simulink model "sampleModel646original"  (R2021b)
settings: Solver=VariableStepAuto  StartTime=0.0  StopTime=10.0  RelTol=1e-3
undefined symbols (not defined in the file): DiscIntNeverNeededParam, Newton, Raphson, sigbuilder_block
libraries: simulink x194, slpidlib x27
(part 3 of 5)

== system sampleModel646original/emi_1578 ==
  In1 : Inport
  emi_1579 : Inport  Port=2
  emi_1581 : DeadZone  SaturateOnIntegerOverflow=on
  emi_1582 : DiscreteIntegrator  SampleTime=-1  ICPrevOutput=DiscIntNeverNeededParam  ICPrevScaledInput=DiscIntNeverNeededParam
  emi_{1583,1595,1598,1600} (4 alike) : simulink/Discontinuities/Saturation Dynamic  OutMin=[]  OutMax=[]  OutDataTypeStr=Inherit: Same as second input  OutDataType=fixdt(1, 16)  OutScaling=2^-10  DoSatur=off
  emi_1584 : Math  SaturateOnIntegerOverflow=on
  emi_1585 : Sqrt  Operator=rSqrt  SaturateOnIntegerOverflow=on
  emi_1586 : simulink/Discontinuities/Rate Limiter Dynamic
  emi_1587 : DiscreteFir
  emi_1588 : MinMax
  emi_1589 : simulink/Discrete/Discrete Derivative  gainval=1.0  ICPrevScaledInput=0.0  OutMin=[]  OutMax=[]  OutDataType=fixdt(1, 16)  OutScaling=2^-10  DoSatur=off
  emi_1590 : DiscreteFir
  emi_1591 : slpidlib/PID Controller  Controller=PID  Form=Parallel  TimeDomain=Discrete-time  UseExternalTs=off  SampleTime=-1  IntegratorMethod=Forward Euler  FilterMethod=Forward Euler  ControllerParametersSource=internal  P=1  I=1  D=0  UseFilter=on  N=100  TunerSelectOption=Transfer Function Based (PID Tuner App)  InitialConditionSource=internal  InitialConditionForIntegrator=0  InitialConditionForFilter=0  DifferentiatorICPrevScaledInput=0  ExternalReset=none  TrackingMode=off  Kt=1  LimitOutput=off  SatLimitsSource=internal  UpperSaturationLimit=inf  LowerSaturationLimit=-inf  LinearizeAsGain=off  AntiWindupMode=none  Kb=1  POutMin=[]  POutMax=[]  IOutMin=[]  IOutMax=[]  DOutMin=[]  DOutMax=[]  NOutMin=[]  NOutMax=[]  SumOutMin=[]  SumOutMax=[]  SaturationOutMin=[]  SaturationOutMax=[]  PParamMin=[]  PParamMax=[]  IParamMin=[]  IParamMax=[]  DParamMin=[]  DParamMax=[]  NParamMin=[]  NParamMax=[]  KbParamMin=[]  KbParamMax=[]  KtParamMin=[]  KtParamMax=[]  KbOutMin=[]  KbOutMax=[]  KtOutMin=[]  KtOutMax=[]  IntegratorOutMin=[]  IntegratorOutMax=[]  FilterOutMin=[]  FilterOutMax=[]  SumI1OutMin=[]  SumI1OutMax=[]  SumI2OutMin=[]  SumI2OutMax=[]  SumI3OutMin=[]  SumI3OutMax=[]  SumI4OutMin=[]  SumI4OutMax=[]  SumDOutMin=[]  SumDOutMax=[]  DifferentiatorOutMin=[]  DifferentiatorOutMax=[]  FilterDiffOutCoefMin=[]  FilterDiffOutCoefMax=[]  ReciprocalOutMin=[]  ReciprocalOutMax=[]  SumDenOutMin=[]  SumDenOutMax=[]  SumNumOutMin=[]  SumNumOutMax=[]  DivideOutMin=[]  DivideOutMax=[]  UdiffTsProdOutMin=[]  UdiffTsProdOutMax=[]  NTsProdOutMin=[]  NTsProdOutMax=[]  UintegralTsProdOutMin=[]  UintegralTsProdOutMax=[]  UngainTsProdOutMin=[]  UngainTsProdOutMax=[]  IntegratorContinuousStateAttributes=''  IntegratorStateMustResolveToSignalObject=off  IntegratorRTWStateStorageClass=Auto  FilterContinuousStateAttributes=''  FilterStateMustResolveToSignalObject=off  FilterRTWStateStorageClass=Auto  ParallelPVariant=InternalParameters  IdealPVariant=Disabled  IVariant=InternalParameters  DVariant=InternalParameters  IntegratorVariant=Discrete  SatVariant=Disabled  AWVariant=Passthrough  PCopyVariant=Disabled  TRVariant=Disabled  FdbkBlocksVariant=Forward  IdealPFdbkVariant=Disabled  SatFdbkVariant=Disabled  DerivativeFilterVariant=ForwardEulerFilter  NVariant=InternalParameters  NCopyVariant=Disabled  FilterICVariant=InternalICsFilter  IntegratorICVariant=InternalICs  ExternalResetVariant=Disabled  TRSumVariant=Passthrough  SumFdbkVariant=Disabled  SumVariant=Sum_PID  TsampFilterVariant=InternalTs  TsampNgainVariant=Passthrough  TsampIntegralVariant=Passthrough  ExternalSaturationOutDataTypeStr=Inherit: Same as second input
  emi_1592 : simulink/Discrete/Difference  ICPrevInput=0.0  OutMin=[]  OutMax=[]  OutDataType=fixdt(1, 16)  OutScaling=2^-10  DoSatur=off
  emi_1593 : Trigonometry
  emi_1594 : Sum  Inputs=+
  emi_1596 : Product  Inputs=*
  emi_1597 : Sum  Inputs=+
  emi_1599 : RateLimiter  SampleTimeMode=inherited
  emi_1601 : DiscreteIntegrator  SampleTime=-1  ICPrevOutput=DiscIntNeverNeededParam  ICPrevScaledInput=DiscIntNeverNeededParam
  emi_1602 : simulink/Discrete/Transfer Fcn First Order  PoleZ=0.95  ICPrevOutput=0.0  DoSatur=off
  emi_1603 : Gain
  emi_1604 : simulink/Discontinuities/Rate Limiter Dynamic
  emi_1605 : DiscreteTransferFcn
  emi_1606 : simulink/Discrete/Discrete Derivative  gainval=1.0  ICPrevScaledInput=0.0  OutMin=[]  OutMax=[]  OutDataType=fixdt(1, 16)  OutScaling=2^-10  DoSatur=off
  emi_1607 : Clock
  Out1 : Outport
  emi_1580 : Outport  Port=2
  wires:
  In1/1 -> Out1/1
  emi_1581/1 -> emi_1582/1
  emi_1582/1 -> emi_1583/1
  emi_1583/1 -> emi_1584/1
  emi_1584/1 -> emi_1585/1
  emi_1585/1 -> emi_1586/1
  emi_1586/1 -> emi_1587/1
  emi_1587/1 -> emi_1588/1
  emi_1588/1 -> emi_1589/1
  emi_1589/1 -> emi_1590/1
  emi_1590/1 -> emi_1591/1
  emi_1591/1 -> emi_1592/1
  emi_1592/1 -> emi_1593/1
  emi_1593/1 -> emi_1594/1
  emi_1594/1 -> emi_1595/1
  emi_1595/1 -> emi_1596/1
  emi_1596/1 -> emi_1597/1
  emi_1597/1 -> emi_1598/1
  emi_1598/1 -> emi_1599/1
  emi_1599/1 -> emi_1600/1
  emi_1600/1 -> emi_1601/1
  emi_1601/1 -> emi_1602/1
  emi_1602/1 -> emi_1603/1
  emi_1603/1 -> emi_1604/1
  emi_1604/1 -> emi_1605/1
  emi_1605/1 -> emi_1606/1
  emi_1607/1 -> emi_1581/1
  emi_1606/1 -> emi_1580/1

== system sampleModel646original/emi_1614 ==
  emi_1621 : Inport
  Action Port : ActionPort  ActionPortLabel=if(0 > u1)
  emi_1618 : Trigonometry  SampleTime=1
  emi_1619 : Gain  SampleTime=1
  emi_1620 : Gain  SampleTime=1
  emi_{1623,1627,1638,1644,1646} (5 alike) : Sin  TimeSource=Use external signal  SampleTime=0
  emi_1624 : Math  SaturateOnIntegerOverflow=on
  emi_1625 : Rounding
  emi_{1626,1632,1640,1642,1650..1651,1653} (7 alike) : Sum  Inputs=+
  emi_1628 : MinMax
  emi_1629 : Sqrt  Operator=rSqrt  SaturateOnIntegerOverflow=on
  emi_1630 : UnaryMinus
  emi_1631 : Product  Inputs=*
  emi_1633 : MinMax
  emi_1634 : Product  Inputs=*
  emi_1635 : Gain
  emi_1636 : Trigonometry
  emi_1637 : Abs
  emi_1639 : Product  Inputs=*
  emi_1641 : Math  SaturateOnIntegerOverflow=on
  emi_1643 : UnaryMinus
  emi_1645 : Trigonometry
  emi_1647 : Rounding
  emi_1648 : Trigonometry
  emi_1649 : MinMax
  emi_1652 : Math  SaturateOnIntegerOverflow=on
  emi_1654 : Sqrt  Operator=rSqrt  SaturateOnIntegerOverflow=on
  emi_1655 : Ground
  emi_1622 : Outport
  wires:
  emi_1621/1 -> emi_1618/1
  emi_1618/1 -> emi_1619/1
  emi_1619/1 -> emi_1620/1
  emi_1623/1 -> emi_1624/1
  emi_1624/1 -> emi_1625/1
  emi_1625/1 -> emi_1626/1
  emi_1626/1 -> emi_1627/1
  emi_1627/1 -> emi_1628/1
  emi_1628/1 -> emi_1629/1
  emi_1629/1 -> emi_1630/1
  emi_1630/1 -> emi_1631/1
  emi_1631/1 -> emi_1632/1
  emi_1632/1 -> emi_1633/1
  emi_1633/1 -> emi_1634/1
  emi_1634/1 -> emi_1635/1
  emi_1635/1 -> emi_1636/1
  emi_1636/1 -> emi_1637/1
  emi_1637/1 -> emi_1638/1
  emi_1638/1 -> emi_1639/1
  emi_1639/1 -> emi_1640/1
  emi_1640/1 -> emi_1641/1
  emi_1641/1 -> emi_1642/1
  emi_1642/1 -> emi_1643/1
  emi_1643/1 -> emi_1644/1
  emi_1644/1 -> emi_1645/1
  emi_1645/1 -> emi_1646/1
  emi_1646/1 -> emi_1647/1
  emi_1647/1 -> emi_1648/1
  emi_1648/1 -> emi_1649/1
  emi_1649/1 -> emi_1650/1
  emi_1650/1 -> emi_1651/1
  emi_1651/1 -> emi_1652/1
  emi_1652/1 -> emi_1653/1
  emi_1653/1 -> emi_1654/1
  emi_1655/1 -> emi_1623/1
  emi_1654/1 -> emi_1622/1

== system sampleModel646original/emi_1658 ==
  In1 : Inport
  emi_1659 : Inport  Port=2
  emi_1661 : Trigonometry
  emi_1662 : Math  SaturateOnIntegerOverflow=on
  emi_1663 : simulink/Discrete/Difference  ICPrevInput=0.0  OutMin=[]  OutMax=[]  OutDataType=fixdt(1, 16)  OutScaling=2^-10  DoSatur=off
  emi_{1664,1679,1682,1691} (4 alike) : simulink/Discrete/Discrete Derivative  gainval=1.0  ICPrevScaledInput=0.0  OutMin=[]  OutMax=[]  OutDataType=fixdt(1, 16)  OutScaling=2^-10  DoSatur=off
  emi_1665 : DiscreteIntegrator  SampleTime=-1  ICPrevOutput=DiscIntNeverNeededParam  ICPrevScaledInput=DiscIntNeverNeededParam
  emi_1666 : RateLimiter  SampleTimeMode=inherited
  emi_1667 : slpidlib/PID Controller  Controller=PID  Form=Parallel  TimeDomain=Discrete-time  UseExternalTs=off  SampleTime=-1  IntegratorMethod=Forward Euler  FilterMethod=Forward Euler  ControllerParametersSource=internal  P=1  I=1  D=0  UseFilter=on  N=100  TunerSelectOption=Transfer Function Based (PID Tuner App)  InitialConditionSource=internal  InitialConditionForIntegrator=0  InitialConditionForFilter=0  DifferentiatorICPrevScaledInput=0  ExternalReset=none  TrackingMode=off  Kt=1  LimitOutput=off  SatLimitsSource=internal  UpperSaturationLimit=inf  LowerSaturationLimit=-inf  LinearizeAsGain=off  AntiWindupMode=none  Kb=1  POutMin=[]  POutMax=[]  IOutMin=[]  IOutMax=[]  DOutMin=[]  DOutMax=[]  NOutMin=[]  NOutMax=[]  SumOutMin=[]  SumOutMax=[]  SaturationOutMin=[]  SaturationOutMax=[]  PParamMin=[]  PParamMax=[]  IParamMin=[]  IParamMax=[]  DParamMin=[]  DParamMax=[]  NParamMin=[]  NParamMax=[]  KbParamMin=[]  KbParamMax=[]  KtParamMin=[]  KtParamMax=[]  KbOutMin=[]  KbOutMax=[]  KtOutMin=[]  KtOutMax=[]  IntegratorOutMin=[]  IntegratorOutMax=[]  FilterOutMin=[]  FilterOutMax=[]  SumI1OutMin=[]  SumI1OutMax=[]  SumI2OutMin=[]  SumI2OutMax=[]  SumI3OutMin=[]  SumI3OutMax=[]  SumI4OutMin=[]  SumI4OutMax=[]  SumDOutMin=[]  SumDOutMax=[]  DifferentiatorOutMin=[]  DifferentiatorOutMax=[]  FilterDiffOutCoefMin=[]  FilterDiffOutCoefMax=[]  ReciprocalOutMin=[]  ReciprocalOutMax=[]  SumDenOutMin=[]  SumDenOutMax=[]  SumNumOutMin=[]  SumNumOutMax=[]  DivideOutMin=[]  DivideOutMax=[]  UdiffTsProdOutMin=[]  UdiffTsProdOutMax=[]  NTsProdOutMin=[]  NTsProdOutMax=[]  UintegralTsProdOutMin=[]  UintegralTsProdOutMax=[]  UngainTsProdOutMin=[]  UngainTsProdOutMax=[]  IntegratorContinuousStateAttributes=''  IntegratorStateMustResolveToSignalObject=off  IntegratorRTWStateStorageClass=Auto  FilterContinuousStateAttributes=''  FilterStateMustResolveToSignalObject=off  FilterRTWStateStorageClass=Auto  ParallelPVariant=InternalParameters  IdealPVariant=Disabled  IVariant=InternalParameters  DVariant=InternalParameters  IntegratorVariant=Discrete  SatVariant=Disabled  AWVariant=Passthrough  PCopyVariant=Disabled  TRVariant=Disabled  FdbkBlocksVariant=Forward  IdealPFdbkVariant=Disabled  SatFdbkVariant=Disabled  DerivativeFilterVariant=ForwardEulerFilter  NVariant=InternalParameters  NCopyVariant=Disabled  FilterICVariant=InternalICsFilter  IntegratorICVariant=InternalICs  ExternalResetVariant=Disabled  TRSumVariant=Passthrough  SumFdbkVariant=Disabled  SumVariant=Sum_PID  TsampFilterVariant=InternalTs  TsampNgainVariant=Passthrough  TsampIntegralVariant=Passthrough  ExternalSaturationOutDataTypeStr=Inherit: Same as second input
  emi_1668 : Sqrt  Operator=rSqrt  SaturateOnIntegerOverflow=on
  emi_1669 : simulink/Discontinuities/Rate Limiter Dynamic
  emi_1670 : slpidlib/PID Controller  Controller=PID  Form=Parallel  TimeDomain=Discrete-time  UseExternalTs=off  SampleTime=-1  IntegratorMethod=Forward Euler  FilterMethod=Forward Euler  ControllerParametersSource=internal  P=1  I=1  D=0  UseFilter=on  N=100  TunerSelectOption=Transfer Function Based (PID Tuner App)  InitialConditionSource=internal  InitialConditionForIntegrator=0  InitialConditionForFilter=0  DifferentiatorICPrevScaledInput=0  ExternalReset=none  TrackingMode=off  Kt=1  LimitOutput=off  SatLimitsSource=internal  UpperSaturationLimit=inf  LowerSaturationLimit=-inf  LinearizeAsGain=off  AntiWindupMode=none  Kb=1  POutMin=[]  POutMax=[]  IOutMin=[]  IOutMax=[]  DOutMin=[]  DOutMax=[]  NOutMin=[]  NOutMax=[]  SumOutMin=[]  SumOutMax=[]  SaturationOutMin=[]  SaturationOutMax=[]  PParamMin=[]  PParamMax=[]  IParamMin=[]  IParamMax=[]  DParamMin=[]  DParamMax=[]  NParamMin=[]  NParamMax=[]  KbParamMin=[]  KbParamMax=[]  KtParamMin=[]  KtParamMax=[]  KbOutMin=[]  KbOutMax=[]  KtOutMin=[]  KtOutMax=[]  IntegratorOutMin=[]  IntegratorOutMax=[]  FilterOutMin=[]  FilterOutMax=[]  SumI1OutMin=[]  SumI1OutMax=[]  SumI2OutMin=[]  SumI2OutMax=[]  SumI3OutMin=[]  SumI3OutMax=[]  SumI4OutMin=[]  SumI4OutMax=[]  SumDOutMin=[]  SumDOutMax=[]  DifferentiatorOutMin=[]  DifferentiatorOutMax=[]  FilterDiffOutCoefMin=[]  FilterDiffOutCoefMax=[]  ReciprocalOutMin=[]  ReciprocalOutMax=[]  SumDenOutMin=[]  SumDenOutMax=[]  SumNumOutMin=[]  SumNumOutMax=[]  DivideOutMin=[]  DivideOutMax=[]  UdiffTsProdOutMin=[]  UdiffTsProdOutMax=[]  NTsProdOutMin=[]  NTsProdOutMax=[]  UintegralTsProdOutMin=[]  UintegralTsProdOutMax=[]  UngainTsProdOutMin=[]  UngainTsProdOutMax=[]  IntegratorContinuousStateAttributes=''  IntegratorStateMustResolveToSignalObject=off  IntegratorRTWStateStorageClass=Auto  FilterContinuousStateAttributes=''  FilterStateMustResolveToSignalObject=off  FilterRTWStateStorageClass=Auto  ParallelPVariant=InternalParameters  IdealPVariant=Disabled  IVariant=InternalParameters  DVariant=InternalParameters  IntegratorVariant=Discrete  SatVariant=Disabled  AWVariant=Passthrough  PCopyVariant=Disabled  TRVariant=Disabled  FdbkBlocksVariant=Forward  IdealPFdbkVariant=Disabled  SatFdbkVariant=Disabled  DerivativeFilterVariant=ForwardEulerFilter  NVariant=InternalParameters  NCopyVariant=Disabled  FilterICVariant=InternalICsFilter  IntegratorICVariant=InternalICs  ExternalResetVariant=Disabled  TRSumVariant=Passthrough  SumFdbkVariant=Disabled  SumVariant=Sum_PID  TsampFilterVariant=InternalTs  TsampNgainVariant=Passthrough  TsampIntegralVariant=Passthrough  ExternalSaturationOutDataTypeStr=Inherit: Same as second input
  emi_1671 : simulink/Discrete/Difference  ICPrevInput=0.0  OutMin=[]  OutMax=[]  OutDataType=fixdt(1, 16)  OutScaling=2^-10  DoSatur=off
  emi_1672 : Math  SaturateOnIntegerOverflow=on
  emi_1673 : Rounding
  emi_1674 : simulink/Discrete/Transfer Fcn First Order  PoleZ=0.95  ICPrevOutput=0.0  DoSatur=off
  emi_1675 : Relay
  emi_1676 : Rounding
  emi_1677 : simulink/Discontinuities/PWM  DisableCoverage=on  Period=1  DisallowZeroDutyCycle=off  RunAtFixedTimeIntervals=off  SampleTime=0.1
  emi_1678 : Sum  Inputs=+
  emi_1680 : simulink/Discontinuities/Saturation Dynamic  OutMin=[]  OutMax=[]  OutDataTypeStr=Inherit: Same as second input  OutDataType=fixdt(1, 16)  OutScaling=2^-10  DoSatur=off
  emi_1681 : Gain
  emi_1683 : RateLimiter  SampleTimeMode=inherited
  emi_1684 : DiscreteFir
  emi_1685 : DeadZone  SaturateOnIntegerOverflow=on
  emi_1686 : simulink/Discontinuities/PWM  DisableCoverage=on  Period=1  DisallowZeroDutyCycle=off  RunAtFixedTimeIntervals=off  SampleTime=0.1
  emi_1687 : Sin  TimeSource=Use external signal  SampleTime=0
  emi_1688 : Quantizer
  emi_1689 : RateLimiter  SampleTimeMode=inherited
  emi_1690 : DiscreteZeroPole  Poles=[0 0.5]  Gain=1  SampleTime=-1
  emi_1692 : simulink/Discontinuities/Wrap To Zero  Threshold=255
      settings: SourceProductBaseCode=SL
  emi_1693 : simulink/Sources/Repeating Sequence  rep_seq_t=[0 2]  rep_seq_y=[0 2]
  Out1 : Outport
  emi_1660 : Outport  Port=2
  wires:
  In1/1 -> Out1/1
  emi_1661/1 -> emi_1662/1
  emi_1662/1 -> emi_1663/1
  emi_1663/1 -> emi_1664/1
  emi_1664/1 -> emi_1665/1
  emi_1665/1 -> emi_1666/1
  emi_1666/1 -> emi_1667/1
  emi_1667/1 -> emi_1668/1
  emi_1668/1 -> emi_1669/1
  emi_1669/1 -> emi_1670/1
  emi_1670/1 -> emi_1671/1
  emi_1671/1 -> emi_1672/1
  emi_1672/1 -> emi_1673/1
  emi_1673/1 -> emi_1674/1
  emi_1674/1 -> emi_1675/1
  emi_1675/1 -> emi_1676/1
  emi_1676/1 -> emi_1677/1
  emi_1677/1 -> emi_1678/1
  emi_1678/1 -> emi_1679/1
  emi_1679/1 -> emi_1680/1
  emi_1680/1 -> emi_1681/1
  emi_1681/1 -> emi_1682/1
  emi_1682/1 -> emi_1683/1
  emi_1683/1 -> emi_1684/1
  emi_1684/1 -> emi_1685/1
  emi_1685/1 -> emi_1686/1
  emi_1686/1 -> emi_1687/1
  emi_1687/1 -> emi_1688/1
  emi_1688/1 -> emi_1689/1
  emi_1689/1 -> emi_1690/1
  emi_1690/1 -> emi_1691/1
  emi_1691/1 -> emi_1692/1
  emi_1693/1 -> emi_1661/1
  emi_1692/1 -> emi_1660/1

== system sampleModel646original/emi_166 ==
  emi_173 : Inport
  Action Port : ActionPort  ActionPortLabel=if(0 > u1)
  emi_170 : MinMax  SampleTime=1
  emi_171 : Trigonometry  SampleTime=1
  emi_172 : Math  SampleTime=1  SaturateOnIntegerOverflow=on
  emi_175 : Trigonometry
  emi_176 : Gain
  emi_177 : Sin  TimeSource=Use external signal  SampleTime=0
  emi_178 : Sqrt  Operator=rSqrt  SaturateOnIntegerOverflow=on
  emi_179 : UnaryMinus
  emi_180 : Sqrt  Operator=rSqrt  SaturateOnIntegerOverflow=on
  emi_181 : Sum  Inputs=+
  emi_182 : MinMax
  emi_183 : Abs
  emi_184 : Sqrt  Operator=rSqrt  SaturateOnIntegerOverflow=on
  emi_185 : Math  SaturateOnIntegerOverflow=on
  emi_186 : UnaryMinus
  emi_187 : UnaryMinus
  emi_188 : Trigonometry
  emi_189 : Rounding
  emi_190 : Math  SaturateOnIntegerOverflow=on
  emi_191 : Gain
  emi_192 : Gain
  emi_193 : Abs
  emi_194 : Ground
  emi_174 : Outport
  wires:
  emi_173/1 -> emi_170/1
  emi_170/1 -> emi_171/1
  emi_171/1 -> emi_172/1
  emi_175/1 -> emi_176/1
  emi_176/1 -> emi_177/1
  emi_177/1 -> emi_178/1
  emi_178/1 -> emi_179/1
  emi_179/1 -> emi_180/1
  emi_180/1 -> emi_181/1
  emi_181/1 -> emi_182/1
  emi_182/1 -> emi_183/1
  emi_183/1 -> emi_184/1
  emi_184/1 -> emi_185/1
  emi_185/1 -> emi_186/1
  emi_186/1 -> emi_187/1
  emi_187/1 -> emi_188/1
  emi_188/1 -> emi_189/1
  emi_189/1 -> emi_190/1
  emi_190/1 -> emi_191/1
  emi_191/1 -> emi_192/1
  emi_192/1 -> emi_193/1
  emi_194/1 -> emi_175/1
  emi_193/1 -> emi_174/1

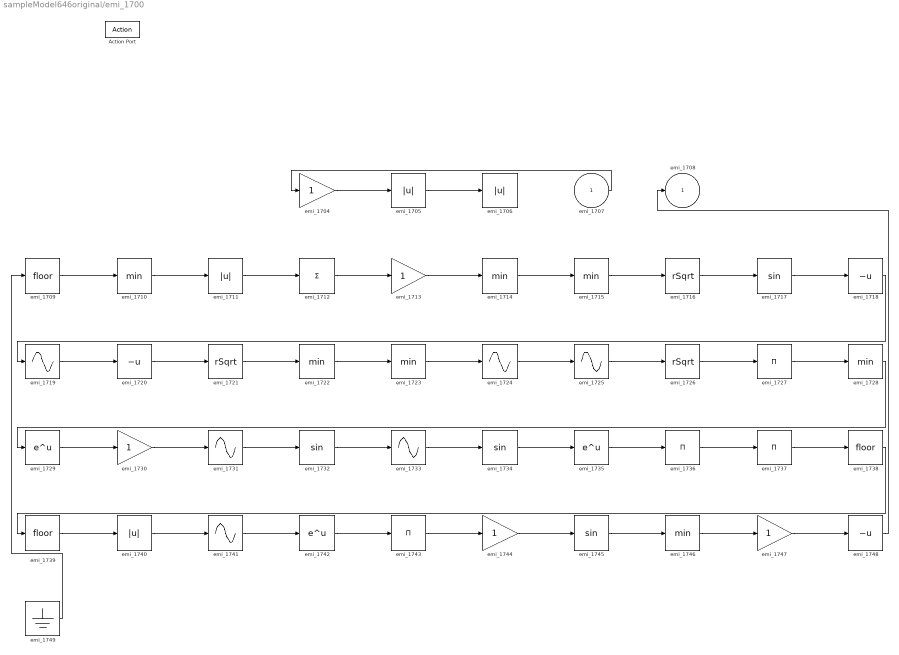
== system sampleModel646original/emi_1700 ==
  emi_1707 : Inport
  Action Port : ActionPort  ActionPortLabel=if(0 > u1)
  emi_{1704,1713,1730,1744,1747} (5 alike) : Gain
  emi_{1705..1706,1711,1740} (4 alike) : Abs
  emi_1709 : Rounding
  emi_{1710,1714..1715,1722..1723,1728,1746} (7 alike) : MinMax
  emi_1712 : Sum  Inputs=+
  emi_1716 : Sqrt  Operator=rSqrt  SaturateOnIntegerOverflow=on
  emi_{1717,1732,1734,1745} (4 alike) : Trigonometry
  emi_1718 : UnaryMinus
  emi_{1719,1724..1725,1731,1733,1741} (6 alike) : Sin  TimeSource=Use external signal  SampleTime=0
  emi_1720 : UnaryMinus
  emi_1721 : Sqrt  Operator=rSqrt  SaturateOnIntegerOverflow=on
  emi_1726 : Sqrt  Operator=rSqrt  SaturateOnIntegerOverflow=on
  emi_{1727,1736..1737,1743} (4 alike) : Product  Inputs=*
  emi_1729 : Math  SaturateOnIntegerOverflow=on
  emi_1735 : Math  SaturateOnIntegerOverflow=on
  emi_1738 : Rounding
  emi_1739 : Rounding
  emi_1742 : Math  SaturateOnIntegerOverflow=on
  emi_1748 : UnaryMinus
  emi_1749 : Ground
  emi_1708 : Outport
  wires:
  emi_1707/1 -> emi_1704/1
  emi_1704/1 -> emi_1705/1
  emi_1705/1 -> emi_1706/1
  emi_1709/1 -> emi_1710/1
  emi_1710/1 -> emi_1711/1
  emi_1711/1 -> emi_1712/1
  emi_1712/1 -> emi_1713/1
  emi_1713/1 -> emi_1714/1
  emi_1714/1 -> emi_1715/1
  emi_1715/1 -> emi_1716/1
  emi_1716/1 -> emi_1717/1
  emi_1717/1 -> emi_1718/1
  emi_1718/1 -> emi_1719/1
  emi_1719/1 -> emi_1720/1
  emi_1720/1 -> emi_1721/1
  emi_1721/1 -> emi_1722/1
  emi_1722/1 -> emi_1723/1
  emi_1723/1 -> emi_1724/1
  emi_1724/1 -> emi_1725/1
  emi_1725/1 -> emi_1726/1
  emi_1726/1 -> emi_1727/1
  emi_1727/1 -> emi_1728/1
  emi_1728/1 -> emi_1729/1
  emi_1729/1 -> emi_1730/1
  emi_1730/1 -> emi_1731/1
  emi_1731/1 -> emi_1732/1
  emi_1732/1 -> emi_1733/1
  emi_1733/1 -> emi_1734/1
  emi_1734/1 -> emi_1735/1
  emi_1735/1 -> emi_1736/1
  emi_1736/1 -> emi_1737/1
  emi_1737/1 -> emi_1738/1
  emi_1738/1 -> emi_1739/1
  emi_1739/1 -> emi_1740/1
  emi_1740/1 -> emi_1741/1
  emi_1741/1 -> emi_1742/1
  emi_1742/1 -> emi_1743/1
  emi_1743/1 -> emi_1744/1
  emi_1744/1 -> emi_1745/1
  emi_1745/1 -> emi_1746/1
  emi_1746/1 -> emi_1747/1
  emi_1747/1 -> emi_1748/1
  emi_1749/1 -> emi_1709/1
  emi_1748/1 -> emi_1708/1

== system sampleModel646original/emi_1752 ==
  In1 : Inport
  emi_1753 : Inport  Port=2
  emi_1755 : simulink/Discontinuities/Saturation Dynamic  OutMin=[]  OutMax=[]  OutDataTypeStr=Inherit: Same as second input  OutDataType=fixdt(1, 16)  OutScaling=2^-10  DoSatur=off
  emi_1756 : Trigonometry
  emi_1757 : simulink/Discontinuities/Rate Limiter Dynamic
  emi_1758 : Trigonometry
  emi_1759 : Sin  TimeSource=Use external signal  SampleTime=0
  emi_1760 : UnaryMinus
  emi_1761 : DiscreteFir
  emi_1762 : Relay
  emi_1763 : simulink/Discontinuities/PWM  DisableCoverage=on  Period=1  DisallowZeroDutyCycle=off  RunAtFixedTimeIntervals=off  SampleTime=0.1
  emi_1764 : simulink/Discontinuities/Wrap To Zero  Threshold=255
      settings: SourceProductBaseCode=SL
  emi_1765 : MinMax
  emi_1766 : Rounding
  emi_1767 : DiscreteStateSpace  SampleTime=-1
  emi_1768 : simulink/Discrete/Transfer Fcn First Order  PoleZ=0.95  ICPrevOutput=0.0  DoSatur=off
  emi_1769 : Quantizer
  emi_1770 : DiscreteTransferFcn
  emi_1771 : simulink/Discontinuities/PWM  DisableCoverage=on  Period=1  DisallowZeroDutyCycle=off  RunAtFixedTimeIntervals=off  SampleTime=0.1
  emi_1772 : simulink/Discontinuities/PWM  DisableCoverage=on  Period=1  DisallowZeroDutyCycle=off  RunAtFixedTimeIntervals=off  SampleTime=0.1
  emi_1773 : DiscretePulseGenerator  PulseType=Time based  Period=10  PulseWidth=5
  Out1 : Outport
  emi_1754 : Outport  Port=2
  wires:
  In1/1 -> Out1/1
  emi_1755/1 -> emi_1756/1
  emi_1756/1 -> emi_1757/1
  emi_1757/1 -> emi_1758/1
  emi_1758/1 -> emi_1759/1
  emi_1759/1 -> emi_1760/1
  emi_1760/1 -> emi_1761/1
  emi_1761/1 -> emi_1762/1
  emi_1762/1 -> emi_1763/1
  emi_1763/1 -> emi_1764/1
  emi_1764/1 -> emi_1765/1
  emi_1765/1 -> emi_1766/1
  emi_1766/1 -> emi_1767/1
  emi_1767/1 -> emi_1768/1
  emi_1768/1 -> emi_1769/1
  emi_1769/1 -> emi_1770/1
  emi_1770/1 -> emi_1771/1
  emi_1771/1 -> emi_1772/1
  emi_1773/1 -> emi_1755/1
  emi_1772/1 -> emi_1754/1

== system sampleModel646original/emi_1781 ==
  emi_1788 : Inport
  Action Port : ActionPort  ActionPortLabel=if(-2 > u1)
  emi_1785 : Gain
  emi_1786 : Gain
  emi_1787 : Math  SaturateOnIntegerOverflow=on
  emi_1790 : UnaryMinus
  emi_1791 : Rounding
  emi_{1792,1795,1798,1801} (4 alike) : Product  Inputs=*
  emi_1793 : Rounding
  emi_1794 : Gain
  emi_1796 : Sin  TimeSource=Use external signal  SampleTime=0
  emi_1797 : Trigonometry
  emi_1799 : Math  SaturateOnIntegerOverflow=on
  emi_1800 : Sqrt  Operator=rSqrt  SaturateOnIntegerOverflow=on
  emi_1802 : UnaryMinus
  emi_1803 : Trigonometry
  emi_1804 : Ground
  emi_1789 : Outport
  wires:
  emi_1788/1 -> emi_1785/1
  emi_1785/1 -> emi_1786/1
  emi_1786/1 -> emi_1787/1
  emi_1790/1 -> emi_1791/1
  emi_1791/1 -> emi_1792/1
  emi_1792/1 -> emi_1793/1
  emi_1793/1 -> emi_1794/1
  emi_1794/1 -> emi_1795/1
  emi_1795/1 -> emi_1796/1
  emi_1796/1 -> emi_1797/1
  emi_1797/1 -> emi_1798/1
  emi_1798/1 -> emi_1799/1
  emi_1799/1 -> emi_1800/1
  emi_1800/1 -> emi_1801/1
  emi_1801/1 -> emi_1802/1
  emi_1802/1 -> emi_1803/1
  emi_1804/1 -> emi_1790/1
  emi_1803/1 -> emi_1789/1

== system sampleModel646original/emi_1807 ==
  In1 : Inport
  emi_1808 : Inport  Port=2
  emi_{1810,1820,1827..1828} (4 alike) : Math  SaturateOnIntegerOverflow=on
  emi_1811 : DiscreteStateSpace  SampleTime=-1
  emi_1812 : DiscreteFir
  emi_1813 : simulink/Discrete/Difference  ICPrevInput=0.0  OutMin=[]  OutMax=[]  OutDataType=fixdt(1, 16)  OutScaling=2^-10  DoSatur=off
  emi_1814 : DeadZone  SaturateOnIntegerOverflow=on
  emi_1815 : VariablePulseGenerator  SampleTime=0.1
  emi_1816 : Sin  TimeSource=Use external signal  SampleTime=0
  emi_1817 : Sqrt  Operator=rSqrt  SaturateOnIntegerOverflow=on
  emi_1818 : Abs
  emi_1819 : DiscreteFir
  emi_1821 : simulink/Discontinuities/Wrap To Zero  Threshold=255
      settings: SourceProductBaseCode=SL
  emi_1822 : simulink/Discontinuities/PWM  DisableCoverage=on  Period=1  DisallowZeroDutyCycle=off  RunAtFixedTimeIntervals=off  SampleTime=0.1
  emi_1823 : DiscreteFir
  emi_1824 : Relay
  emi_1825 : Abs
  emi_1826 : Relay
  emi_1829 : slpidlib/PID Controller  Controller=PID  Form=Parallel  TimeDomain=Discrete-time  UseExternalTs=off  SampleTime=-1  IntegratorMethod=Forward Euler  FilterMethod=Forward Euler  ControllerParametersSource=internal  P=1  I=1  D=0  UseFilter=on  N=100  TunerSelectOption=Transfer Function Based (PID Tuner App)  InitialConditionSource=internal  InitialConditionForIntegrator=0  InitialConditionForFilter=0  DifferentiatorICPrevScaledInput=0  ExternalReset=none  TrackingMode=off  Kt=1  LimitOutput=off  SatLimitsSource=internal  UpperSaturationLimit=inf  LowerSaturationLimit=-inf  LinearizeAsGain=off  AntiWindupMode=none  Kb=1  POutMin=[]  POutMax=[]  IOutMin=[]  IOutMax=[]  DOutMin=[]  DOutMax=[]  NOutMin=[]  NOutMax=[]  SumOutMin=[]  SumOutMax=[]  SaturationOutMin=[]  SaturationOutMax=[]  PParamMin=[]  PParamMax=[]  IParamMin=[]  IParamMax=[]  DParamMin=[]  DParamMax=[]  NParamMin=[]  NParamMax=[]  KbParamMin=[]  KbParamMax=[]  KtParamMin=[]  KtParamMax=[]  KbOutMin=[]  KbOutMax=[]  KtOutMin=[]  KtOutMax=[]  IntegratorOutMin=[]  IntegratorOutMax=[]  FilterOutMin=[]  FilterOutMax=[]  SumI1OutMin=[]  SumI1OutMax=[]  SumI2OutMin=[]  SumI2OutMax=[]  SumI3OutMin=[]  SumI3OutMax=[]  SumI4OutMin=[]  SumI4OutMax=[]  SumDOutMin=[]  SumDOutMax=[]  DifferentiatorOutMin=[]  DifferentiatorOutMax=[]  FilterDiffOutCoefMin=[]  FilterDiffOutCoefMax=[]  ReciprocalOutMin=[]  ReciprocalOutMax=[]  SumDenOutMin=[]  SumDenOutMax=[]  SumNumOutMin=[]  SumNumOutMax=[]  DivideOutMin=[]  DivideOutMax=[]  UdiffTsProdOutMin=[]  UdiffTsProdOutMax=[]  NTsProdOutMin=[]  NTsProdOutMax=[]  UintegralTsProdOutMin=[]  UintegralTsProdOutMax=[]  UngainTsProdOutMin=[]  UngainTsProdOutMax=[]  IntegratorContinuousStateAttributes=''  IntegratorStateMustResolveToSignalObject=off  IntegratorRTWStateStorageClass=Auto  FilterContinuousStateAttributes=''  FilterStateMustResolveToSignalObject=off  FilterRTWStateStorageClass=Auto  ParallelPVariant=InternalParameters  IdealPVariant=Disabled  IVariant=InternalParameters  DVariant=InternalParameters  IntegratorVariant=Discrete  SatVariant=Disabled  AWVariant=Passthrough  PCopyVariant=Disabled  TRVariant=Disabled  FdbkBlocksVariant=Forward  IdealPFdbkVariant=Disabled  SatFdbkVariant=Disabled  DerivativeFilterVariant=ForwardEulerFilter  NVariant=InternalParameters  NCopyVariant=Disabled  FilterICVariant=InternalICsFilter  IntegratorICVariant=InternalICs  ExternalResetVariant=Disabled  TRSumVariant=Passthrough  SumFdbkVariant=Disabled  SumVariant=Sum_PID  TsampFilterVariant=InternalTs  TsampNgainVariant=Passthrough  TsampIntegralVariant=Passthrough  ExternalSaturationOutDataTypeStr=Inherit: Same as second input
  emi_1830 : slpidlib/PID Controller  Controller=PID  Form=Parallel  TimeDomain=Discrete-time  UseExternalTs=off  SampleTime=-1  IntegratorMethod=Forward Euler  FilterMethod=Forward Euler  ControllerParametersSource=internal  P=1  I=1  D=0  UseFilter=on  N=100  TunerSelectOption=Transfer Function Based (PID Tuner App)  InitialConditionSource=internal  InitialConditionForIntegrator=0  InitialConditionForFilter=0  DifferentiatorICPrevScaledInput=0  ExternalReset=none  TrackingMode=off  Kt=1  LimitOutput=off  SatLimitsSource=internal  UpperSaturationLimit=inf  LowerSaturationLimit=-inf  LinearizeAsGain=off  AntiWindupMode=none  Kb=1  POutMin=[]  POutMax=[]  IOutMin=[]  IOutMax=[]  DOutMin=[]  DOutMax=[]  NOutMin=[]  NOutMax=[]  SumOutMin=[]  SumOutMax=[]  SaturationOutMin=[]  SaturationOutMax=[]  PParamMin=[]  PParamMax=[]  IParamMin=[]  IParamMax=[]  DParamMin=[]  DParamMax=[]  NParamMin=[]  NParamMax=[]  KbParamMin=[]  KbParamMax=[]  KtParamMin=[]  KtParamMax=[]  KbOutMin=[]  KbOutMax=[]  KtOutMin=[]  KtOutMax=[]  IntegratorOutMin=[]  IntegratorOutMax=[]  FilterOutMin=[]  FilterOutMax=[]  SumI1OutMin=[]  SumI1OutMax=[]  SumI2OutMin=[]  SumI2OutMax=[]  SumI3OutMin=[]  SumI3OutMax=[]  SumI4OutMin=[]  SumI4OutMax=[]  SumDOutMin=[]  SumDOutMax=[]  DifferentiatorOutMin=[]  DifferentiatorOutMax=[]  FilterDiffOutCoefMin=[]  FilterDiffOutCoefMax=[]  ReciprocalOutMin=[]  ReciprocalOutMax=[]  SumDenOutMin=[]  SumDenOutMax=[]  SumNumOutMin=[]  SumNumOutMax=[]  DivideOutMin=[]  DivideOutMax=[]  UdiffTsProdOutMin=[]  UdiffTsProdOutMax=[]  NTsProdOutMin=[]  NTsProdOutMax=[]  UintegralTsProdOutMin=[]  UintegralTsProdOutMax=[]  UngainTsProdOutMin=[]  UngainTsProdOutMax=[]  IntegratorContinuousStateAttributes=''  IntegratorStateMustResolveToSignalObject=off  IntegratorRTWStateStorageClass=Auto  FilterContinuousStateAttributes=''  FilterStateMustResolveToSignalObject=off  FilterRTWStateStorageClass=Auto  ParallelPVariant=InternalParameters  IdealPVariant=Disabled  IVariant=InternalParameters  DVariant=InternalParameters  IntegratorVariant=Discrete  SatVariant=Disabled  AWVariant=Passthrough  PCopyVariant=Disabled  TRVariant=Disabled  FdbkBlocksVariant=Forward  IdealPFdbkVariant=Disabled  SatFdbkVariant=Disabled  DerivativeFilterVariant=ForwardEulerFilter  NVariant=InternalParameters  NCopyVariant=Disabled  FilterICVariant=InternalICsFilter  IntegratorICVariant=InternalICs  ExternalResetVariant=Disabled  TRSumVariant=Passthrough  SumFdbkVariant=Disabled  SumVariant=Sum_PID  TsampFilterVariant=InternalTs  TsampNgainVariant=Passthrough  TsampIntegralVariant=Passthrough  ExternalSaturationOutDataTypeStr=Inherit: Same as second input
  emi_1831 : Product  Inputs=*
  emi_1832 : Quantizer
  emi_1833 : Abs
  emi_1834 : Sum  Inputs=+
  emi_1835 : simulink/Sources/Chirp Signal  f1=0.1  T=100  f2=1
  Out1 : Outport
  emi_1809 : Outport  Port=2
  wires:
  In1/1 -> Out1/1
  emi_1810/1 -> emi_1811/1
  emi_1811/1 -> emi_1812/1
  emi_1812/1 -> emi_1813/1
  emi_1813/1 -> emi_1814/1
  emi_1814/1 -> emi_1815/1
  emi_1815/1 -> emi_1816/1
  emi_1816/1 -> emi_1817/1
  emi_1817/1 -> emi_1818/1
  emi_1818/1 -> emi_1819/1
  emi_1819/1 -> emi_1820/1
  emi_1820/1 -> emi_1821/1
  emi_1821/1 -> emi_1822/1
  emi_1822/1 -> emi_1823/1
  emi_1823/1 -> emi_1824/1
  emi_1824/1 -> emi_1825/1
  emi_1825/1 -> emi_1826/1
  emi_1826/1 -> emi_1827/1
  emi_1827/1 -> emi_1828/1
  emi_1828/1 -> emi_1829/1
  emi_1829/1 -> emi_1830/1
  emi_1830/1 -> emi_1831/1
  emi_1831/1 -> emi_1832/1
  emi_1832/1 -> emi_1833/1
  emi_1833/1 -> emi_1834/1
  emi_1835/1 -> emi_1810/1
  emi_1834/1 -> emi_1809/1

== system sampleModel646original/emi_1842 ==
  emi_1849 : Inport
  Action Port : ActionPort  ActionPortLabel=if(0 > u1)
  emi_1846 : Abs
  emi_1847 : Math  SaturateOnIntegerOverflow=on
  emi_1848 : Gain
  emi_1851 : Abs
  emi_{1852,1860..1862} (4 alike) : Trigonometry
  emi_1853 : UnaryMinus
  emi_1854 : Product  Inputs=*
  emi_1855 : MinMax
  emi_1856 : Sqrt  Operator=rSqrt  SaturateOnIntegerOverflow=on
  emi_1857 : Sum  Inputs=+
  emi_1858 : Gain
  emi_1859 : Sin  TimeSource=Use external signal  SampleTime=0
  emi_1863 : Rounding
  emi_1864 : Ground
  emi_1850 : Outport
  wires:
  emi_1849/1 -> emi_1846/1
  emi_1846/1 -> emi_1847/1
  emi_1847/1 -> emi_1848/1
  emi_1851/1 -> emi_1852/1
  emi_1852/1 -> emi_1853/1
  emi_1853/1 -> emi_1854/1
  emi_1854/1 -> emi_1855/1
  emi_1855/1 -> emi_1856/1
  emi_1856/1 -> emi_1857/1
  emi_1857/1 -> emi_1858/1
  emi_1858/1 -> emi_1859/1
  emi_1859/1 -> emi_1860/1
  emi_1860/1 -> emi_1861/1
  emi_1861/1 -> emi_1862/1
  emi_1862/1 -> emi_1863/1
  emi_1864/1 -> emi_1851/1
  emi_1863/1 -> emi_1850/1

== system sampleModel646original/emi_1867 ==
  In1 : Inport
  emi_1868 : Inport  Port=2
  emi_1870 : Sum  Inputs=+
  emi_1871 : Sqrt  Operator=rSqrt  SaturateOnIntegerOverflow=on
  emi_1872 : slpidlib/PID Controller  Controller=PID  Form=Parallel  TimeDomain=Discrete-time  UseExternalTs=off  SampleTime=-1  IntegratorMethod=Forward Euler  FilterMethod=Forward Euler  ControllerParametersSource=internal  P=1  I=1  D=0  UseFilter=on  N=100  TunerSelectOption=Transfer Function Based (PID Tuner App)  InitialConditionSource=internal  InitialConditionForIntegrator=0  InitialConditionForFilter=0  DifferentiatorICPrevScaledInput=0  ExternalReset=none  TrackingMode=off  Kt=1  LimitOutput=off  SatLimitsSource=internal  UpperSaturationLimit=inf  LowerSaturationLimit=-inf  LinearizeAsGain=off  AntiWindupMode=none  Kb=1  POutMin=[]  POutMax=[]  IOutMin=[]  IOutMax=[]  DOutMin=[]  DOutMax=[]  NOutMin=[]  NOutMax=[]  SumOutMin=[]  SumOutMax=[]  SaturationOutMin=[]  SaturationOutMax=[]  PParamMin=[]  PParamMax=[]  IParamMin=[]  IParamMax=[]  DParamMin=[]  DParamMax=[]  NParamMin=[]  NParamMax=[]  KbParamMin=[]  KbParamMax=[]  KtParamMin=[]  KtParamMax=[]  KbOutMin=[]  KbOutMax=[]  KtOutMin=[]  KtOutMax=[]  IntegratorOutMin=[]  IntegratorOutMax=[]  FilterOutMin=[]  FilterOutMax=[]  SumI1OutMin=[]  SumI1OutMax=[]  SumI2OutMin=[]  SumI2OutMax=[]  SumI3OutMin=[]  SumI3OutMax=[]  SumI4OutMin=[]  SumI4OutMax=[]  SumDOutMin=[]  SumDOutMax=[]  DifferentiatorOutMin=[]  DifferentiatorOutMax=[]  FilterDiffOutCoefMin=[]  FilterDiffOutCoefMax=[]  ReciprocalOutMin=[]  ReciprocalOutMax=[]  SumDenOutMin=[]  SumDenOutMax=[]  SumNumOutMin=[]  SumNumOutMax=[]  DivideOutMin=[]  DivideOutMax=[]  UdiffTsProdOutMin=[]  UdiffTsProdOutMax=[]  NTsProdOutMin=[]  NTsProdOutMax=[]  UintegralTsProdOutMin=[]  UintegralTsProdOutMax=[]  UngainTsProdOutMin=[]  UngainTsProdOutMax=[]  IntegratorContinuousStateAttributes=''  IntegratorStateMustResolveToSignalObject=off  IntegratorRTWStateStorageClass=Auto  FilterContinuousStateAttributes=''  FilterStateMustResolveToSignalObject=off  FilterRTWStateStorageClass=Auto  ParallelPVariant=InternalParameters  IdealPVariant=Disabled  IVariant=InternalParameters  DVariant=InternalParameters  IntegratorVariant=Discrete  SatVariant=Disabled  AWVariant=Passthrough  PCopyVariant=Disabled  TRVariant=Disabled  FdbkBlocksVariant=Forward  IdealPFdbkVariant=Disabled  SatFdbkVariant=Disabled  DerivativeFilterVariant=ForwardEulerFilter  NVariant=InternalParameters  NCopyVariant=Disabled  FilterICVariant=InternalICsFilter  IntegratorICVariant=InternalICs  ExternalResetVariant=Disabled  TRSumVariant=Passthrough  SumFdbkVariant=Disabled  SumVariant=Sum_PID  TsampFilterVariant=InternalTs  TsampNgainVariant=Passthrough  TsampIntegralVariant=Passthrough  ExternalSaturationOutDataTypeStr=Inherit: Same as second input
  emi_1873 : Quantizer
  emi_1874 : VariablePulseGenerator  SampleTime=0.1
  emi_1875 : Product  Inputs=*
  emi_1876 : VariablePulseGenerator  SampleTime=0.1
  emi_1877 : simulink/Discontinuities/Rate Limiter Dynamic
  emi_1878 : DiscreteFilter
  emi_1879 : DiscreteIntegrator  SampleTime=-1  ICPrevOutput=DiscIntNeverNeededParam  ICPrevScaledInput=DiscIntNeverNeededParam
  emi_1880 : VariablePulseGenerator  SampleTime=0.1
  emi_1881 : Math  SaturateOnIntegerOverflow=on
  emi_1882 : MinMax
  emi_1883 : DiscreteFir
  emi_1884 : DiscreteZeroPole  Poles=[0 0.5]  Gain=1  SampleTime=-1
  emi_1885 : Trigonometry
  emi_1886 : DiscreteZeroPole  Poles=[0 0.5]  Gain=1  SampleTime=-1
  emi_1887 : SignalGenerator  Units=rad/sec
  Out1 : Outport
  emi_1869 : Outport  Port=2
  wires:
  In1/1 -> Out1/1
  emi_1870/1 -> emi_1871/1
  emi_1871/1 -> emi_1872/1
  emi_1872/1 -> emi_1873/1
  emi_1873/1 -> emi_1874/1
  emi_1874/1 -> emi_1875/1
  emi_1875/1 -> emi_1876/1
  emi_1876/1 -> emi_1877/1
  emi_1877/1 -> emi_1878/1
  emi_1878/1 -> emi_1879/1
  emi_1879/1 -> emi_1880/1
  emi_1880/1 -> emi_1881/1
  emi_1881/1 -> emi_1882/1
  emi_1882/1 -> emi_1883/1
  emi_1883/1 -> emi_1884/1
  emi_1884/1 -> emi_1885/1
  emi_1885/1 -> emi_1886/1
  emi_1887/1 -> emi_1870/1
  emi_1886/1 -> emi_1869/1

== system sampleModel646original/emi_1894 ==
  emi_1901 : Inport
  Action Port : ActionPort  ActionPortLabel=if(0 > u1)
  emi_1898 : Gain
  emi_1899 : Math  SaturateOnIntegerOverflow=on
  emi_{1900,1906,1911,1913,1916} (5 alike) : MinMax
  emi_1903 : Trigonometry
  emi_1904 : Sqrt  Operator=rSqrt  SaturateOnIntegerOverflow=on
  emi_1905 : Sin  TimeSource=Use external signal  SampleTime=0
  emi_1907 : Sin  TimeSource=Use external signal  SampleTime=0
  emi_1908 : Sum  Inputs=+
  emi_1909 : Product  Inputs=*
  emi_1910 : UnaryMinus
  emi_1912 : Abs
  emi_1914 : Sqrt  Operator=rSqrt  SaturateOnIntegerOverflow=on
  emi_1915 : Math  SaturateOnIntegerOverflow=on
  emi_1917 : Ground
  emi_1902 : Outport
  wires:
  emi_1901/1 -> emi_1898/1
  emi_1898/1 -> emi_1899/1
  emi_1899/1 -> emi_1900/1
  emi_1903/1 -> emi_1904/1
  emi_1904/1 -> emi_1905/1
  emi_1905/1 -> emi_1906/1
  emi_1906/1 -> emi_1907/1
  emi_1907/1 -> emi_1908/1
  emi_1908/1 -> emi_1909/1
  emi_1909/1 -> emi_1910/1
  emi_1910/1 -> emi_1911/1
  emi_1911/1 -> emi_1912/1
  emi_1912/1 -> emi_1913/1
  emi_1913/1 -> emi_1914/1
  emi_1914/1 -> emi_1915/1
  emi_1915/1 -> emi_1916/1
  emi_1917/1 -> emi_1903/1
  emi_1916/1 -> emi_1902/1

== system sampleModel646original/emi_1920 ==
  In1 : Inport
  emi_1921 : Inport  Port=2
  emi_1923 : MinMax
  emi_1924 : Sum  Inputs=+
  emi_1925 : RateLimiter  SampleTimeMode=inherited
  emi_1926 : simulink/Discrete/Transfer Fcn First Order  PoleZ=0.95  ICPrevOutput=0.0  DoSatur=off
  emi_1927 : Relay
  emi_1928 : simulink/Discontinuities/Wrap To Zero  Threshold=255
      settings: SourceProductBaseCode=SL
  emi_1929 : RateLimiter  SampleTimeMode=inherited
  emi_1930 : simulink/Discontinuities/Saturation Dynamic  OutMin=[]  OutMax=[]  OutDataTypeStr=Inherit: Same as second input  OutDataType=fixdt(1, 16)  OutScaling=2^-10  DoSatur=off
  emi_1931 : Quantizer
  emi_1932 : MinMax
  emi_1933 : DiscreteTransferFcn
  emi_1934 : UnaryMinus
  emi_1935 : DiscretePulseGenerator  PulseType=Time based  Period=10  PulseWidth=5
  Out1 : Outport
  emi_1922 : Outport  Port=2
  wires:
  In1/1 -> Out1/1
  emi_1923/1 -> emi_1924/1
  emi_1924/1 -> emi_1925/1
  emi_1925/1 -> emi_1926/1
  emi_1926/1 -> emi_1927/1
  emi_1927/1 -> emi_1928/1
  emi_1928/1 -> emi_1929/1
  emi_1929/1 -> emi_1930/1
  emi_1930/1 -> emi_1931/1
  emi_1931/1 -> emi_1932/1
  emi_1932/1 -> emi_1933/1
  emi_1933/1 -> emi_1934/1
  emi_1935/1 -> emi_1923/1
  emi_1934/1 -> emi_1922/1

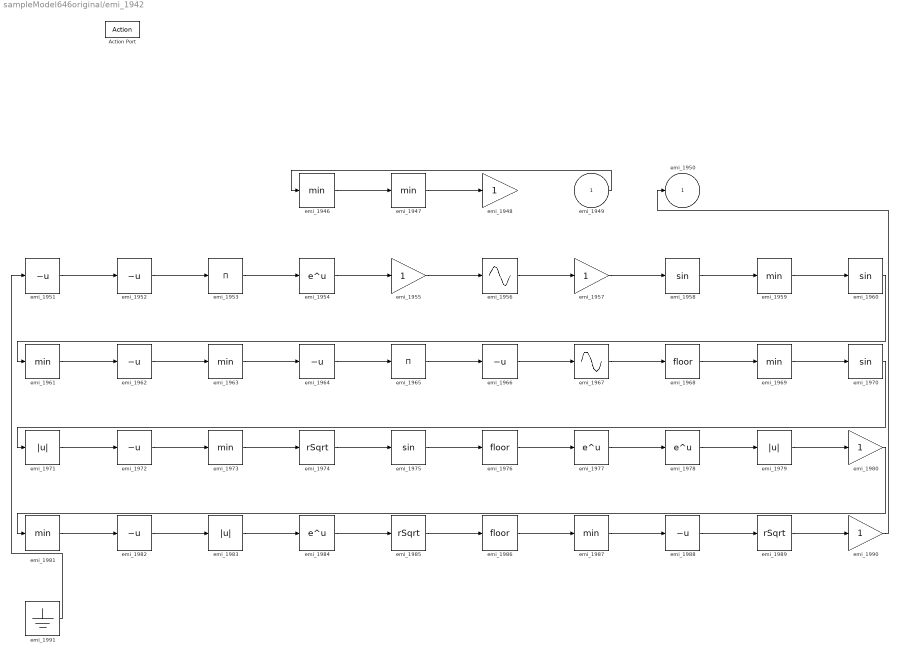
== system sampleModel646original/emi_1942 ==
  emi_1949 : Inport
  Action Port : ActionPort  ActionPortLabel=if(0 > u1)
  emi_{1946..1947,1959,1961,1963,1969,1973,1981,1987} (9 alike) : MinMax
  emi_{1948,1955,1957,1980,1990} (5 alike) : Gain
  emi_{1951..1952,1962,1964,1966,1972,1982,1988} (8 alike) : UnaryMinus
  emi_1953 : Product  Inputs=*
  emi_{1954,1977..1978,1984} (4 alike) : Math  SaturateOnIntegerOverflow=on
  emi_1956 : Sin  TimeSource=Use external signal  SampleTime=0
  emi_{1958,1960,1970,1975} (4 alike) : Trigonometry
  emi_1965 : Product  Inputs=*
  emi_1967 : Sin  TimeSource=Use external signal  SampleTime=0
  emi_1968 : Rounding
  emi_1971 : Abs
  emi_1974 : Sqrt  Operator=rSqrt  SaturateOnIntegerOverflow=on
  emi_1976 : Rounding
  emi_1979 : Abs
  emi_1983 : Abs
  emi_1985 : Sqrt  Operator=rSqrt  SaturateOnIntegerOverflow=on
  emi_1986 : Rounding
  emi_1989 : Sqrt  Operator=rSqrt  SaturateOnIntegerOverflow=on
  emi_1991 : Ground
  emi_1950 : Outport
  wires:
  emi_1949/1 -> emi_1946/1
  emi_1946/1 -> emi_1947/1
  emi_1947/1 -> emi_1948/1
  emi_1951/1 -> emi_1952/1
  emi_1952/1 -> emi_1953/1
  emi_1953/1 -> emi_1954/1
  emi_1954/1 -> emi_1955/1
  emi_1955/1 -> emi_1956/1
  emi_1956/1 -> emi_1957/1
  emi_1957/1 -> emi_1958/1
  emi_1958/1 -> emi_1959/1
  emi_1959/1 -> emi_1960/1
  emi_1960/1 -> emi_1961/1
  emi_1961/1 -> emi_1962/1
  emi_1962/1 -> emi_1963/1
  emi_1963/1 -> emi_1964/1
  emi_1964/1 -> emi_1965/1
  emi_1965/1 -> emi_1966/1
  emi_1966/1 -> emi_1967/1
  emi_1967/1 -> emi_1968/1
  emi_1968/1 -> emi_1969/1
  emi_1969/1 -> emi_1970/1
  emi_1970/1 -> emi_1971/1
  emi_1971/1 -> emi_1972/1
  emi_1972/1 -> emi_1973/1
  emi_1973/1 -> emi_1974/1
  emi_1974/1 -> emi_1975/1
  emi_1975/1 -> emi_1976/1
  emi_1976/1 -> emi_1977/1
  emi_1977/1 -> emi_1978/1
  emi_1978/1 -> emi_1979/1
  emi_1979/1 -> emi_1980/1
  emi_1980/1 -> emi_1981/1
  emi_1981/1 -> emi_1982/1
  emi_1982/1 -> emi_1983/1
  emi_1983/1 -> emi_1984/1
  emi_1984/1 -> emi_1985/1
  emi_1985/1 -> emi_1986/1
  emi_1986/1 -> emi_1987/1
  emi_1987/1 -> emi_1988/1
  emi_1988/1 -> emi_1989/1
  emi_1989/1 -> emi_1990/1
  emi_1991/1 -> emi_1951/1
  emi_1990/1 -> emi_1950/1

== system sampleModel646original/emi_197 ==
  In1 : Inport
  emi_198 : Inport  Port=2
  emi_200 : Quantizer
  emi_201 : DeadZone  SaturateOnIntegerOverflow=on
  emi_202 : Sqrt  Operator=rSqrt  SaturateOnIntegerOverflow=on
  emi_203 : DiscreteFir
  emi_204 : simulink/Sources/Repeating Sequence Stair  OutValues=[3 1 4 2 1].'  tsamp=-1  OutMin=[]  OutMax=[]  OutDataTypeStr=double  OutputDataTypeScalingMode=double  OutDataType=fixdt(0,8)  ConRadixGroup=Best Precision: Vector-wise  OutScaling=2^-12
  Out1 : Outport
  emi_199 : Outport  Port=2
  wires:
  In1/1 -> Out1/1
  emi_200/1 -> emi_201/1
  emi_201/1 -> emi_202/1
  emi_202/1 -> emi_203/1
  emi_204/1 -> emi_200/1
  emi_203/1 -> emi_199/1

== system sampleModel646original/emi_1994 ==
  In1 : Inport
  emi_1995 : Inport  Port=2
  emi_1997 : Sum  Inputs=+
  emi_1998 : Sin  TimeSource=Use external signal  SampleTime=0
  emi_1999 : DiscreteStateSpace  SampleTime=-1
  emi_2000 : Trigonometry
  emi_2001 : RateLimiter  SampleTimeMode=inherited
  emi_2002 : DiscreteZeroPole  Poles=[0 0.5]  Gain=1  SampleTime=-1
  emi_2003 : VariablePulseGenerator  SampleTime=0.1
  emi_2004 : simulink/Discrete/Discrete Derivative  gainval=1.0  ICPrevScaledInput=0.0  OutMin=[]  OutMax=[]  OutDataType=fixdt(1, 16)  OutScaling=2^-10  DoSatur=off
  emi_2005 : Sqrt  Operator=rSqrt  SaturateOnIntegerOverflow=on
  emi_2006 : simulink/Discontinuities/PWM  DisableCoverage=on  Period=1  DisallowZeroDutyCycle=off  RunAtFixedTimeIntervals=off  SampleTime=0.1
  emi_2007 : simulink/Discrete/Discrete Derivative  gainval=1.0  ICPrevScaledInput=0.0  OutMin=[]  OutMax=[]  OutDataType=fixdt(1, 16)  OutScaling=2^-10  DoSatur=off
  emi_2008 : Sqrt  Operator=rSqrt  SaturateOnIntegerOverflow=on
  emi_2009 : MinMax
  emi_2010 : MinMax
  emi_2011 : simulink/Sources/Band-Limited White Noise  Cov=[0.1]  Ts=0.1  seed=[23341]
  Out1 : Outport
  emi_1996 : Outport  Port=2
  wires:
  In1/1 -> Out1/1
  emi_1997/1 -> emi_1998/1
  emi_1998/1 -> emi_1999/1
  emi_1999/1 -> emi_2000/1
  emi_2000/1 -> emi_2001/1
  emi_2001/1 -> emi_2002/1
  emi_2002/1 -> emi_2003/1
  emi_2003/1 -> emi_2004/1
  emi_2004/1 -> emi_2005/1
  emi_2005/1 -> emi_2006/1
  emi_2006/1 -> emi_2007/1
  emi_2007/1 -> emi_2008/1
  emi_2008/1 -> emi_2009/1
  emi_2009/1 -> emi_2010/1
  emi_2011/1 -> emi_1997/1
  emi_2010/1 -> emi_1996/1

== system sampleModel646original/emi_2018 ==
  emi_2025 : Inport
  Action Port : ActionPort  ActionPortLabel=if(0 > u1)
  emi_{2022,2028,2033,2043} (4 alike) : Trigonometry
  emi_{2023..2024,2027,2035,2037} (5 alike) : MinMax
  emi_2029 : Gain
  emi_2030 : Abs
  emi_2031 : Sqrt  Operator=rSqrt  SaturateOnIntegerOverflow=on
  emi_2032 : Rounding
  emi_2034 : Gain
  emi_2036 : Sum  Inputs=+
  emi_2038 : Gain
  emi_2039 : Sqrt  Operator=rSqrt  SaturateOnIntegerOverflow=on
  emi_{2040..2042,2046} (4 alike) : Math  SaturateOnIntegerOverflow=on
  emi_2044 : Sum  Inputs=+
  emi_2045 : Sum  Inputs=+
  emi_2047 : Abs
  emi_2048 : Ground
  emi_2026 : Outport
  wires:
  emi_2025/1 -> emi_2022/1
  emi_2022/1 -> emi_2023/1
  emi_2023/1 -> emi_2024/1
  emi_2027/1 -> emi_2028/1
  emi_2028/1 -> emi_2029/1
  emi_2029/1 -> emi_2030/1
  emi_2030/1 -> emi_2031/1
  emi_2031/1 -> emi_2032/1
  emi_2032/1 -> emi_2033/1
  emi_2033/1 -> emi_2034/1
  emi_2034/1 -> emi_2035/1
  emi_2035/1 -> emi_2036/1
  emi_2036/1 -> emi_2037/1
  emi_2037/1 -> emi_2038/1
  emi_2038/1 -> emi_2039/1
  emi_2039/1 -> emi_2040/1
  emi_2040/1 -> emi_2041/1
  emi_2041/1 -> emi_2042/1
  emi_2042/1 -> emi_2043/1
  emi_2043/1 -> emi_2044/1
  emi_2044/1 -> emi_2045/1
  emi_2045/1 -> emi_2046/1
  emi_2046/1 -> emi_2047/1
  emi_2048/1 -> emi_2027/1
  emi_2047/1 -> emi_2026/1

== system sampleModel646original/emi_2051 ==
  In1 : Inport
  emi_2052 : Inport  Port=2
  emi_2054 : Relay
  emi_2055 : Sum  Inputs=+
  emi_2056 : simulink/Discrete/Difference  ICPrevInput=0.0  OutMin=[]  OutMax=[]  OutDataType=fixdt(1, 16)  OutScaling=2^-10  DoSatur=off
  emi_2057 : simulink/Discrete/Transfer Fcn First Order  PoleZ=0.95  ICPrevOutput=0.0  DoSatur=off
  emi_2058 : Sqrt  Operator=rSqrt  SaturateOnIntegerOverflow=on
  emi_2059 : Relay
  emi_2060 : Product  Inputs=*
  emi_2061 : Sin  TimeSource=Use external signal  SampleTime=0
  emi_2062 : MinMax
  emi_2063 : Gain
  emi_2064 : Quantizer
  emi_2065 : Sum  Inputs=+
  emi_2066 : simulink/Discontinuities/Wrap To Zero  Threshold=255
      settings: SourceProductBaseCode=SL
  emi_2067 : simulink/Discrete/Transfer Fcn First Order  PoleZ=0.95  ICPrevOutput=0.0  DoSatur=off
  emi_2068 : DiscreteZeroPole  Poles=[0 0.5]  Gain=1  SampleTime=-1
  emi_2069 : Math  SaturateOnIntegerOverflow=on
  emi_2070 : SignalGenerator  Units=rad/sec
  Out1 : Outport
  emi_2053 : Outport  Port=2
  wires:
  In1/1 -> Out1/1
  emi_2054/1 -> emi_2055/1
  emi_2055/1 -> emi_2056/1
  emi_2056/1 -> emi_2057/1
  emi_2057/1 -> emi_2058/1
  emi_2058/1 -> emi_2059/1
  emi_2059/1 -> emi_2060/1
  emi_2060/1 -> emi_2061/1
  emi_2061/1 -> emi_2062/1
  emi_2062/1 -> emi_2063/1
  emi_2063/1 -> emi_2064/1
  emi_2064/1 -> emi_2065/1
  emi_2065/1 -> emi_2066/1
  emi_2066/1 -> emi_2067/1
  emi_2067/1 -> emi_2068/1
  emi_2068/1 -> emi_2069/1
  emi_2070/1 -> emi_2054/1
  emi_2069/1 -> emi_2053/1

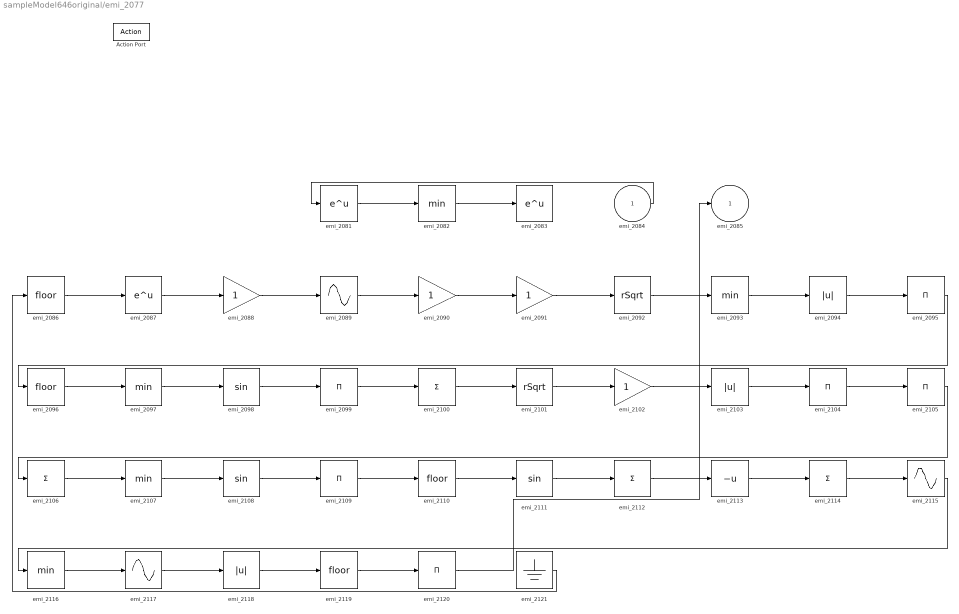
== system sampleModel646original/emi_2077 ==
  emi_2084 : Inport
  Action Port : ActionPort  ActionPortLabel=if(0 > u1)
  emi_2081 : Math  SaturateOnIntegerOverflow=on
  emi_{2082,2093,2097,2107,2116} (5 alike) : MinMax
  emi_2083 : Math  SaturateOnIntegerOverflow=on
  emi_{2086,2096,2110,2119} (4 alike) : Rounding
  emi_2087 : Math  SaturateOnIntegerOverflow=on
  emi_{2088,2090..2091,2102} (4 alike) : Gain
  emi_2089 : Sin  TimeSource=Use external signal  SampleTime=0
  emi_2092 : Sqrt  Operator=rSqrt  SaturateOnIntegerOverflow=on
  emi_2094 : Abs
  emi_{2095,2099,2104..2105,2109,2120} (6 alike) : Product  Inputs=*
  emi_2098 : Trigonometry
  emi_{2100,2106,2112,2114} (4 alike) : Sum  Inputs=+
  emi_2101 : Sqrt  Operator=rSqrt  SaturateOnIntegerOverflow=on
  emi_2103 : Abs
  emi_2108 : Trigonometry
  emi_2111 : Trigonometry
  emi_2113 : UnaryMinus
  emi_2115 : Sin  TimeSource=Use external signal  SampleTime=0
  emi_2117 : Sin  TimeSource=Use external signal  SampleTime=0
  emi_2118 : Abs
  emi_2121 : Ground
  emi_2085 : Outport
  wires:
  emi_2084/1 -> emi_2081/1
  emi_2081/1 -> emi_2082/1
  emi_2082/1 -> emi_2083/1
  emi_2086/1 -> emi_2087/1
  emi_2087/1 -> emi_2088/1
  emi_2088/1 -> emi_2089/1
  emi_2089/1 -> emi_2090/1
  emi_2090/1 -> emi_2091/1
  emi_2091/1 -> emi_2092/1
  emi_2092/1 -> emi_2093/1
  emi_2093/1 -> emi_2094/1
  emi_2094/1 -> emi_2095/1
  emi_2095/1 -> emi_2096/1
  emi_2096/1 -> emi_2097/1
  emi_2097/1 -> emi_2098/1
  emi_2098/1 -> emi_2099/1
  emi_2099/1 -> emi_2100/1
  emi_2100/1 -> emi_2101/1
  emi_2101/1 -> emi_2102/1
  emi_2102/1 -> emi_2103/1
  emi_2103/1 -> emi_2104/1
  emi_2104/1 -> emi_2105/1
  emi_2105/1 -> emi_2106/1
  emi_2106/1 -> emi_2107/1
  emi_2107/1 -> emi_2108/1
  emi_2108/1 -> emi_2109/1
  emi_2109/1 -> emi_2110/1
  emi_2110/1 -> emi_2111/1
  emi_2111/1 -> emi_2112/1
  emi_2112/1 -> emi_2113/1
  emi_2113/1 -> emi_2114/1
  emi_2114/1 -> emi_2115/1
  emi_2115/1 -> emi_2116/1
  emi_2116/1 -> emi_2117/1
  emi_2117/1 -> emi_2118/1
  emi_2118/1 -> emi_2119/1
  emi_2119/1 -> emi_2120/1
  emi_2121/1 -> emi_2086/1
  emi_2120/1 -> emi_2085/1

== system sampleModel646original/emi_211 ==
  emi_218 : Inport
  Action Port : ActionPort  ActionPortLabel=if(0 > u1)
  emi_215 : Abs  SampleTime=1
  emi_216 : MinMax  SampleTime=1
  emi_217 : MinMax  SampleTime=1
  emi_220 : Gain
  emi_221 : Gain
  emi_222 : Sin  TimeSource=Use external signal  SampleTime=0
  emi_223 : Gain
  emi_224 : Product  Inputs=*
  emi_225 : Product  Inputs=*
  emi_226 : Sum  Inputs=+
  emi_227 : UnaryMinus
  emi_228 : Ground
  emi_219 : Outport
  wires:
  emi_218/1 -> emi_215/1
  emi_215/1 -> emi_216/1
  emi_216/1 -> emi_217/1
  emi_220/1 -> emi_221/1
  emi_221/1 -> emi_222/1
  emi_222/1 -> emi_223/1
  emi_223/1 -> emi_224/1
  emi_224/1 -> emi_225/1
  emi_225/1 -> emi_226/1
  emi_226/1 -> emi_227/1
  emi_228/1 -> emi_220/1
  emi_227/1 -> emi_219/1
